simulink model "modelLba3"  (R2021a)
settings: Solver=VariableStepAuto  StartTime=0.0  StopTime=10.0  RelTol=1e-3
values from neighbouring files (symbols this model uses):
  J = 0.0023    [RunModel.m]
  K_d = 0.25    [RunModel.m]
  k_e = 0.274    [RunModel.m]
  K_i = 0.01    [RunModel.m]
  k_m = k_e    (= 0.274)    [RunModel.m]
  K_p = 5    [RunModel.m]
  L = 0.0047    [RunModel.m]
  M_oth = 0.25    [RunModel.m]
  R_electronic = 4.73    [RunModel.m]
  target = 360    [RunModel.m]
  U_max = 7.02    [RunModel.m]
libraries: pid_lib x1
settings Model: Creator=Admin  LastModifiedBy=Admin

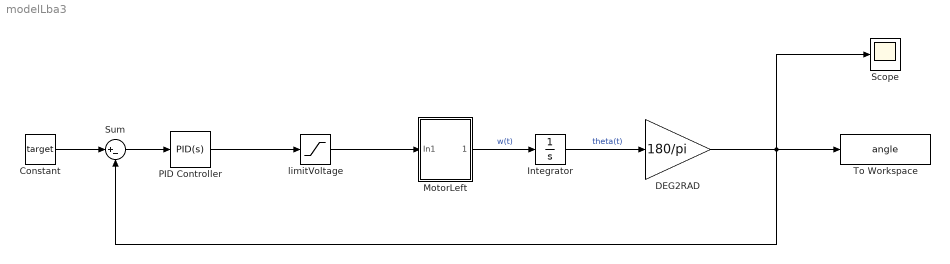
== system modelLba3 ==
  Constant : Constant  Value=target
  DEG2RAD : Gain  Gain=180/pi
  Integrator : Integrator
  MotorLeft : Subsystem
  PID Controller : pid_lib/PID Controller  Controller=PID  Form=Parallel  TimeDomain=Continuous-time  UseExternalTs=off  SampleTime=-1  IntegratorMethod=Forward Euler  FilterMethod=Forward Euler  ControllerParametersSource=internal  P=K_p  I=K_i  D=K_d  UseFilter=on  N=100  TunerSelectOption=Transfer Function Based (PID Tuner App)  InitialConditionSource=internal  InitialConditionForIntegrator=0  InitialConditionForFilter=0  DifferentiatorICPrevScaledInput=0  ExternalReset=none  TrackingMode=off  Kt=1  LimitOutput=off  SatLimitsSource=internal  UpperSaturationLimit=inf  LowerSaturationLimit=-inf  LinearizeAsGain=on  AntiWindupMode=none  Kb=1  POutMin=[]  POutMax=[]  IOutMin=[]  IOutMax=[]  DOutMin=[]  DOutMax=[]  NOutMin=[]  NOutMax=[]  SumOutMin=[]  SumOutMax=[]  SaturationOutMin=[]  SaturationOutMax=[]  PParamMin=[]  PParamMax=[]  IParamMin=[]  IParamMax=[]  DParamMin=[]  DParamMax=[]  NParamMin=[]  NParamMax=[]  KbParamMin=[]  KbParamMax=[]  KtParamMin=[]  KtParamMax=[]  KbOutMin=[]  KbOutMax=[]  KtOutMin=[]  KtOutMax=[]  IntegratorOutMin=[]  IntegratorOutMax=[]  FilterOutMin=[]  FilterOutMax=[]  SumI1OutMin=[]  SumI1OutMax=[]  SumI2OutMin=[]  SumI2OutMax=[]  SumI3OutMin=[]  SumI3OutMax=[]  SumI4OutMin=[]  SumI4OutMax=[]  SumDOutMin=[]  SumDOutMax=[]  DifferentiatorOutMin=[]  DifferentiatorOutMax=[]  FilterDiffOutCoefMin=[]  FilterDiffOutCoefMax=[]  ReciprocalOutMin=[]  ReciprocalOutMax=[]  SumDenOutMin=[]  SumDenOutMax=[]  SumNumOutMin=[]  SumNumOutMax=[]  DivideOutMin=[]  DivideOutMax=[]  UdiffTsProdOutMin=[]  UdiffTsProdOutMax=[]  NTsProdOutMin=[]  NTsProdOutMax=[]  UintegralTsProdOutMin=[]  UintegralTsProdOutMax=[]  UngainTsProdOutMin=[]  UngainTsProdOutMax=[]  IntegratorContinuousStateAttributes=''  IntegratorStateMustResolveToSignalObject=off  IntegratorRTWStateStorageClass=Auto  FilterContinuousStateAttributes=''  FilterStateMustResolveToSignalObject=off  FilterRTWStateStorageClass=Auto  ParallelPVariant=InternalParameters  IdealPVariant=Disabled  IVariant=InternalParameters  DVariant=InternalParameters  IntegratorVariant=Continuous  SatVariant=Disabled  AWVariant=Passthrough  PCopyVariant=Disabled  TRVariant=Disabled  FdbkBlocksVariant=Forward  IdealPFdbkVariant=Disabled  SatFdbkVariant=Disabled  DerivativeFilterVariant=ContFilter  NVariant=InternalParameters  NCopyVariant=Disabled  FilterICVariant=InternalICsFilter  IntegratorICVariant=InternalICs  ExternalResetVariant=Disabled  TRSumVariant=Passthrough  SumFdbkVariant=Disabled  SumVariant=Sum_PID  TsampFilterVariant=InternalTs  TsampNgainVariant=Passthrough  TsampIntegralVariant=Passthrough  ExternalSaturationOutDataTypeStr=Inherit: Same as second input
  Scope : Scope
  Sum : Sum  Inputs=|+-
  To Workspace : ToWorkspace  VariableName=angle  SaveFormat=Timeseries  SampleTime=-1
  limitVoltage : Saturate  UpperLimit=100  LowerLimit=-100
  wires:
  PID Controller/1 -> limitVoltage/1
  limitVoltage/1 -> MotorLeft/1(In1)
  MotorLeft/1(Output) -> Integrator/1  "w(t)"
  Constant/1 -> Sum/1
  Sum/1 -> PID Controller/1
  Integrator/1 -> DEG2RAD/1  "theta(t)"
  DEG2RAD/1 -> Scope/1, Sum/2, To Workspace/1

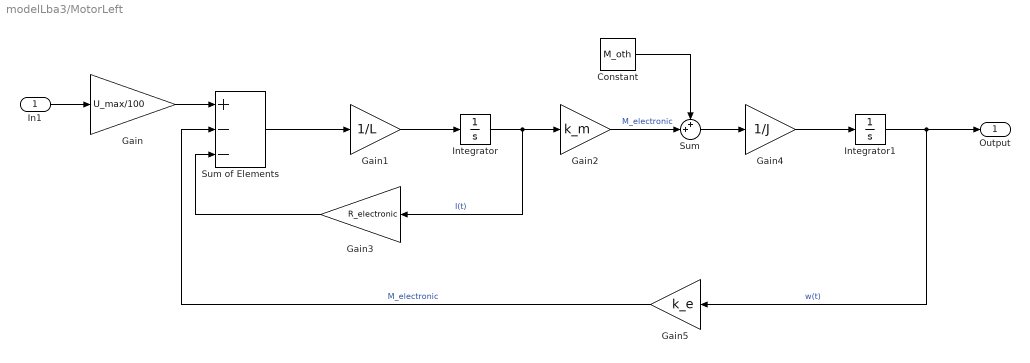
== system modelLba3/MotorLeft ==
  In1 : Inport
  Constant : Constant  Value=M_oth
  Gain : Gain  Gain=U_max/100
  Gain1 : Gain  Gain=1/L
  Gain2 : Gain  Gain=k_m
  Gain3 : Gain  Gain=R_electronic
  Gain4 : Gain  Gain=1/J
  Gain5 : Gain  Gain=k_e
  Integrator : Integrator
  Integrator1 : Integrator
  Sum : Sum  Inputs=++|
  Sum of Elements : Sum  Inputs=+--
  Output : Outport
  wires:
  Gain1/1 -> Integrator/1
  Integrator/1 -> Gain3/1, Gain2/1  "I(t)"
  Constant/1 -> Sum/1
  Sum/1 -> Gain4/1
  Gain/1 -> Sum of Elements/1
  Gain2/1 -> Sum/2  "M_electronic"
  Sum of Elements/1 -> Gain1/1
  Gain5/1 -> Sum of Elements/2  "M_electronic"
  Gain4/1 -> Integrator1/1
  Gain3/1 -> Sum of Elements/3
  Integrator1/1 -> Output/1, Gain5/1  "w(t)"
  In1/1 -> Gain/1
